simulink model "Q1Sim"  (R2022a)
settings: Solver=FixedStepAuto  StartTime=0.0  StopTime=2  FixedStep=0.001  RelTol=1e-3
values from neighbouring files (symbols this model uses):
  A = [0 0 1; 0 0 0; 92.8581 0 0]    [Q1C.m]    (also in Q1Gustavo.m = double(subs(jacobian(f),[x1 x2],[0 0])))
  B = [0; 1; -79.361]    [Q1C.m]    (also in Q1Gustavo.m = double(subs(u,[x1 x2],[0 0])))
  C = [1 0 0]    [Q1C.m]    (also in Q1Gustavo.m)
  D = zeros(3,1)    [Q1C.m]    (also in Q1Gustavo.m = 0)
  K1 = acker(A,B,P1)    [Q1Gustavo.m]
  K2 = place(A,B,P2)    [Q1Gustavo.m]
  x0 = [pi/3 0 0]    [Q1C.m]
settings Model: Creator=Crippa  LastModifiedBy=Crippa
settings SolverCC: ZeroCrossControl=DisableAll

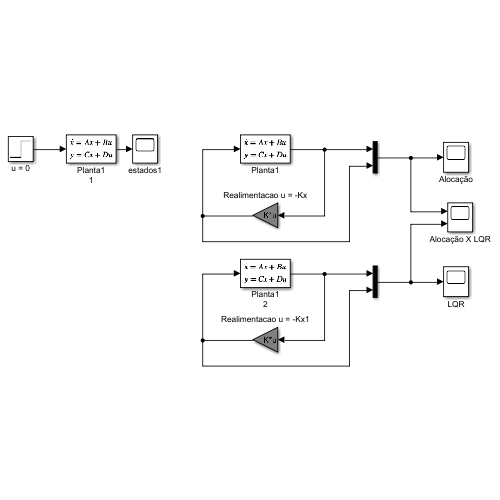
[thumbnail: Simulink's stored preview of the top-level diagram]
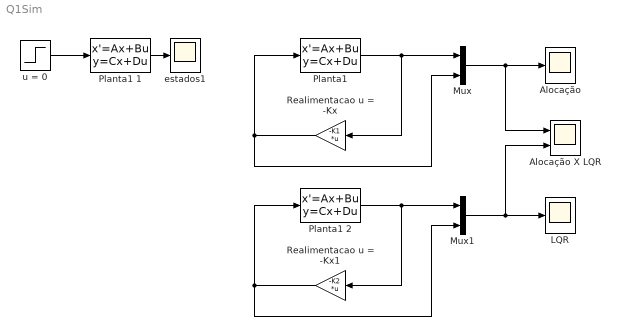
== system Q1Sim ==
  Alocação : Scope
  Alocação X LQR : Scope  NumInputPorts=2
  LQR : Scope
  Mux : Mux  Inputs=2
  Mux1 : Mux  Inputs=2
  "Planta1 " : StateSpace  A=A  B=B  C=C  D=D  InitialCondition=x0
  Planta1 1 : StateSpace  A=A  B=B  C=C  D=D  InitialCondition=x0
  Planta1 2 : StateSpace  A=A  B=B  C=C  D=D  InitialCondition=x0
  Realimentacao u = -Kx : Gain  Gain=-K1  Multiplication=Matrix(K*u)
  Realimentacao u = -Kx1 : Gain  Gain=-K2  Multiplication=Matrix(K*u)
  estados1 : Scope
  u = 0 : Step  Time=0  After=0  SampleTime=0
  wires:
  "Planta1 "/1 -> Mux/1, Realimentacao u = -Kx/1
  Realimentacao u = -Kx/1 -> "Planta1 "/1, Mux/2
  Mux/1 -> Alocação/1, Alocação X LQR/1
  u = 0/1 -> Planta1 1/1
  Planta1 1/1 -> estados1/1
  Planta1 2/1 -> Mux1/1, Realimentacao u = -Kx1/1
  Realimentacao u = -Kx1/1 -> Planta1 2/1, Mux1/2
  Mux1/1 -> Alocação X LQR/2, LQR/1
